simulink model "Bai_2_matlab"  (R2017b)
settings: Solver=FixedStepAuto  StartTime=0.0  StopTime=10  FixedStep=0.01  RelTol=1e-3
values from neighbouring files (symbols this model uses):
  A = [ 0 1 0 0; 10.78 0 0 0; 0 0 0 1; -0.98 0 0 0]    [LQG_dienKalman.m]
  B = [0; -1 ; 0; 1]    [LQG_dienKalman.m]
  C = [1 0 0 0; 0 0 1 0]    [LQG_dienKalman.m]
  K = lqr(A,B,Q,R)    [LQG_dienKalman.m]
  L = lqe(A,G,C,Qn,Rn)    [LQG_dienKalman.m]
  theta_init = pi/18    (= 0.174532925199)    [LQG_dienKalman.m]
  thetadot_init = 0    [LQG_dienKalman.m]
  x_init = 0    [LQG_dienKalman.m]
  xdot_init = 0    [LQG_dienKalman.m]
settings Model: Creator=kinge  LastModifiedBy=ADMIN

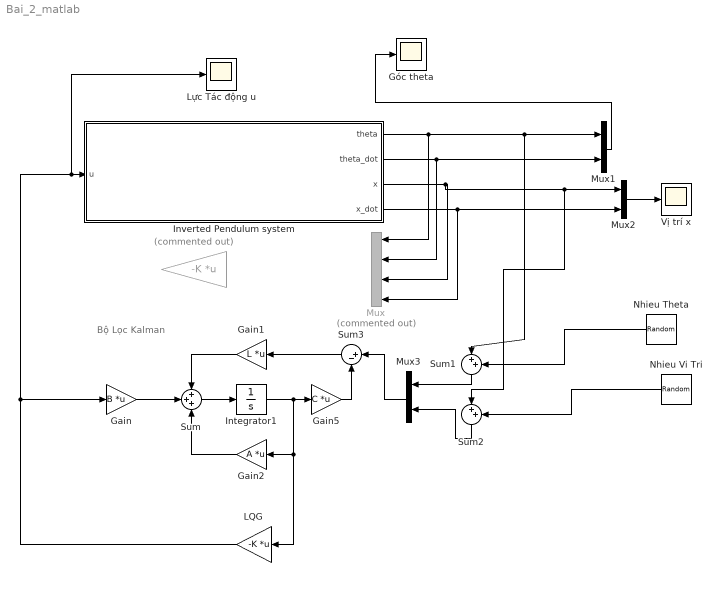
== system Bai_2_matlab ==
  note: Bộ Lọc Kalman
  "  " : Gain  Commented=on  Gain=-K  Multiplication=Matrix(K*u) (u vector)
  "  LQG" : Gain  Gain=-K  Multiplication=Matrix(K*u)
  Gain : Gain  Gain=B  Multiplication=Matrix(K*u)
  Gain1 : Gain  Gain=L  Multiplication=Matrix(K*u)
  Gain2 : Gain  Gain=A  Multiplication=Matrix(K*u)
  Gain5 : Gain  Gain=C  Multiplication=Matrix(K*u)
  Góc theta : Scope
  Integrator1 : Integrator
  Inverted Pendulum system : Subsystem
      settings: MinAlgLoopOccurrences=on
  Lực Tác động u : Scope
  Mux : Mux  Commented=on
  Mux1 : Mux  Inputs=2
  Mux2 : Mux  Inputs=2
  Mux3 : Mux  Inputs=2
  "Nhieu Theta " : RandomNumber  Variance=0.001  SampleTime=0.01
  Nhieu Vi Tri : RandomNumber  Variance=0.01  SampleTime=0.01
  Sum : Sum  Inputs=+++
  Sum1 : Sum  Inputs=|++
  Sum2 : Sum  Inputs=|++
  Sum3 : Sum  Inputs=|+-
  Vị trí x : Scope
  wires:
  Mux2/1 -> Vị trí x/1
  Mux1/1 -> Góc theta/1
  Inverted Pendulum system/2(theta_dot) -> Mux1/2, Mux/2
  Inverted Pendulum system/4(x_dot) -> Mux2/2, Mux/4
  Gain/1 -> Sum/2
  Sum/1 -> Integrator1/1
  Gain1/1 -> Sum/1
  Gain2/1 -> Sum/3
  Integrator1/1 -> "  LQG"/1, Gain2/1, Gain5/1
  Gain5/1 -> Sum3/2
  Sum3/1 -> Gain1/1
  Inverted Pendulum system/1("theta ") -> Mux/1, Mux1/1, Sum1/1
  Mux3/1 -> Sum3/1
  Inverted Pendulum system/3(x) -> Sum2/1, Mux2/1, Mux/3
  "Nhieu Theta "/1 -> Sum1/2
  Nhieu Vi Tri/1 -> Sum2/2
  Sum1/1 -> Mux3/1
  Sum2/1 -> Mux3/2
  "  LQG"/1 -> Gain/1, Lực Tác động u/1, Inverted Pendulum system/1("u ")

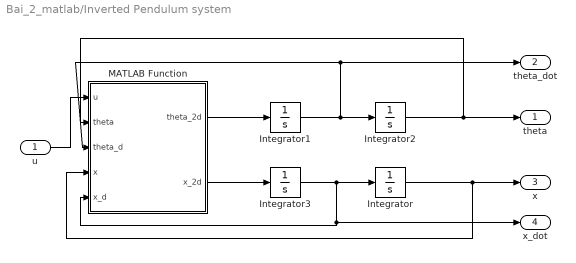
== system Bai_2_matlab/Inverted Pendulum system ==
  "u " : Inport
  Integrator : Integrator  InitialCondition=xdot_init
  Integrator1 : Integrator  InitialCondition=theta_init
  Integrator2 : Integrator  InitialCondition=thetadot_init
  Integrator3 : Integrator  InitialCondition=x_init
  MATLAB Function : MATLAB Function  TreatAsAtomicUnit=on
  "theta " : Outport
  theta_dot : Outport  Port=2
  x : Outport  Port=3
  x_dot : Outport  Port=4
  wires:
  Integrator3/1 -> MATLAB Function/5(x_d), x_dot/1, Integrator/1
  Integrator/1 -> MATLAB Function/4(x), x/1
  "u "/1 -> MATLAB Function/1(u)
  Integrator1/1 -> theta_dot/1, MATLAB Function/3(theta_d), Integrator2/1
  Integrator2/1 -> MATLAB Function/2(theta), "theta "/1
  MATLAB Function/1(theta_2d) -> Integrator1/1
  MATLAB Function/2(x_2d) -> Integrator3/1

== matlab function Bai_2_matlab/Inverted Pendulum system/MATLAB Function ==
  data: u input; theta input; theta_d input; theta_2d output; x_2d output; x input; x_d input
function [theta_2d, x_2d] = Inverted_Pendulum(u, theta, theta_d, x, x_d)
%% Declaration
M = 1;
m = 0.1;
l = 1;
g = 9.81;

%% Simulink he con lac nguoc
x_2d = (u + m*l*sin(theta)*(theta_d)^2 - m*g*cos(theta)*sin(theta)) / (M + m - m*(cos(theta))^2);
theta_2d = ((u*cos(theta) - (M + m)*g*sin(theta) + m*l*cos(theta)*sin(theta)*(theta_d)^2)) /(m*l*(cos(theta))^2 - (M + m)*l);
